simulink model "white_noise_whistle3"  (Simulink 7.3)
settings: Solver=ode3  StartTime=0.0  StopTime=1  FixedStep=1/11025  MaxStep=1/11025  MinStep=1/11025  RelTol=1e-3
libraries: simulink x1, simulink_extras x1
settings Model: Creator=Hörnstein  LastModifiedBy=Hörnstein
settings SolverCC: InitialStep=1/11025
settings OptimizationCC: InitFltsAndDblsToZero=on
settings DebuggingCC: AlgebraicLoopMsg=none  SaveWithParameterizedLinksMsg=none  SignalResolutionControl=TryResolveAllWithWarning  MultiTaskDSMMsg=warning  MultiTaskCondExecSysMsg=none
settings RTWCC: IncludeERTFirstTime=on
settings GRTTargetCC: TargetFcnLib=ansi_tfl_tmw.mat

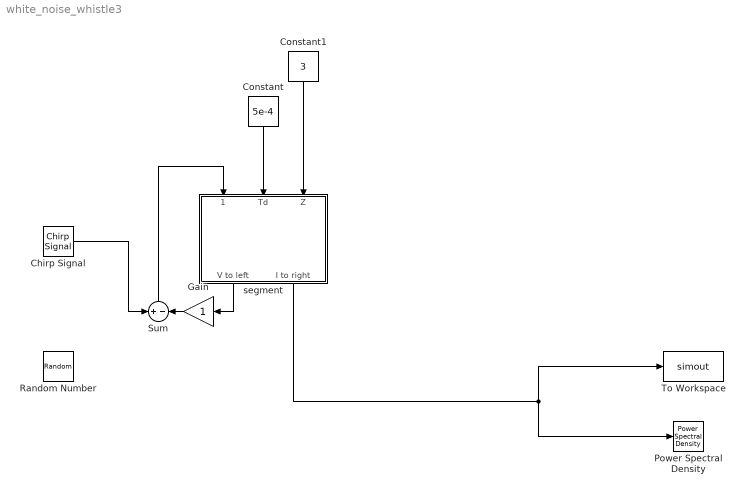
== system white_noise_whistle3 ==
  Chirp Signal : simulink/Sources/Chirp Signal  SystemSampleTime=-1  f1=0  T=1  f2=2000
  Constant : Constant  Value=5e-4  OutDataType=sfix(16)  OutScaling=2^0
  Constant1 : Constant  Value=3  OutDataType=sfix(16)  OutScaling=2^0
  Gain : Gain  ParameterDataType=sfix(16)  ParameterScaling=2^0  OutDataType=sfix(16)  OutScaling=2^0
  Power Spectral Density : simulink_extras/Additional Sinks/Power Spectral Density  SystemSampleTime=-1  npts=1102  fftpts=1102  HowOften=64  sampleT=1/11025
  Random Number : RandomNumber  SampleTime=0
  Sum : Sum  Inputs=+|-  OutDataType=sfix(16)  OutScaling=2^0
  To Workspace : ToWorkspace  VariableName=simout  SampleTime=-1  SaveFormat=Array
  segment : Subsystem
  wires:
  Constant/1 -> segment/2(Td)
  Constant1/1 -> segment/3(Z)
  Sum/1 -> segment/1(I from left)
  Gain/1 -> Sum/2
  Chirp Signal/1 -> Sum/1
  segment/2(I to right) -> To Workspace/1, Power Spectral Density/1
  segment/1(V to left) -> Gain/1

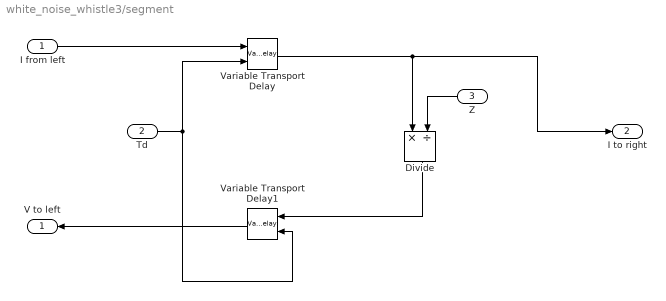
== system white_noise_whistle3/segment ==
  I from left : Inport  OutDataType=sfix(16)  OutScaling=2^0
  Td : Inport  Port=2  OutDataType=sfix(16)  OutScaling=2^0
  Z : Inport  Port=3  OutDataType=sfix(16)  OutScaling=2^0
  Divide : Product  Inputs=*/  OutDataType=sfix(16)  OutScaling=2^-10
  Variable Transport Delay : VariableTransportDelay  VariableDelayType=Variable transport delay  MaximumDelay=10
  Variable Transport Delay1 : VariableTransportDelay  VariableDelayType=Variable transport delay  MaximumDelay=10
  V to left : Outport  OutDataType=sfix(16)  OutScaling=2^0
  I to right : Outport  Port=2  OutDataType=sfix(16)  OutScaling=2^0
  wires:
  Variable Transport Delay1/1 -> V to left/1
  Z/1 -> Divide/2
  Variable Transport Delay/1 -> Divide/1, I to right/1
  I from left/1 -> Variable Transport Delay/1
  Td/1 -> Variable Transport Delay/2, Variable Transport Delay1/2
  Divide/1 -> Variable Transport Delay1/1
